simulink model "gm_flyback_pid_vnl"  (R2021b)
settings: Solver=FixedStepDiscrete  StartTime=0.0  StopTime=100e-3  RelTol=1e-3
undefined symbols (not defined in the file or in its folder): DiscIntNeverNeededParam
libraries: simulink x6
Description:
  | Symmetric FIR Filter
  | This example shows how to use HDL Coder(TM) to check, generate,
  | and verify HDL for a fixed-point symmetric FIR filter.
settings Model: Creator=The MathWorks, Inc.  LastModifiedBy=Marco Milanesi
settings SolverCC: AlgebraicLoopSolver=TrustRegion  AutoInsertRateTranBlk=on
settings DataIOCC: LimitDataPoints=on  SaveFormat=Array  SaveOutput=off  SignalLogging=off  SaveTime=off  ReturnWorkspaceOutputs=off  SignalLoggingName=logsOut
settings OptimizationCC: BlockReduction=off  BooleanDataType=off  ConditionallyExecuteInputs=off  DefaultParameterBehavior=Inlined  InheritOutputTypeSmallerThanSingle=on  InlineInvariantSignals=on  ExpressionDepthLimit=2147483647  InitFltsAndDblsToZero=on  LifeSpan=inf  BufferReusableBoundary=off
settings DebuggingCC: AlgebraicLoopMsg=error  SaveWithParameterizedLinksMsg=none  UnderspecifiedInitializationDetection=Classic  MergeDetectMultiDrivingBlocksExec=none  CheckExecutionContextPreStartOutputMsg=on  SignalResolutionControl=TryResolveAllWithWarning  InheritedTsInSrcMsg=none  MultiTaskDSMMsg=warning  MultiTaskCondExecSysMsg=none  SingleTaskRateTransMsg=error  IntegerOverflowMsg=none  ParameterPrecisionLossMsg=none  FcnCallInpInsideContextMsg=warning  BusObjectLabelMismatch=none  StateNameClashWarn=warning  SFUnexpectedBacktrackingDiag=warning  SFNoUnconditionalDefaultTransitionDiag=warning  SFExecutionAtInitializationDiag=none  SFMachineParentedDataDiag=warning  IntegerSaturationMsg=none  ArithmeticOperatorsInVariantConditions=warning
settings HardwareCC: ProdBitPerPointer=32  ProdBitPerSizeT=32  ProdBitPerPtrDiffT=32  ProdLargestAtomicFloat=None  ProdIntDivRoundTo=Undefined  ProdEndianess=Unspecified  ProdWordSize=32  ProdHWDeviceType=ASIC/FPGA  TargetUnknown=on  ProdEqTarget=off
settings ModelReferenceCC: PropagateSignalLabelsOutOfModel=off
settings SFSimCC: SimUseLocalCustomCode=off  CustomCodeUndefinedFunction=UseInterfaceOnly
settings RTWCC: RTWUseLocalCustomCode=off
settings CodeAppCC: StateflowObjectComments=on
settings GRTTargetCC: TargetFcnLib=ansi_tfl_tmw.mat  TargetLangStandard=C89/C90 (ANSI)  CombineOutputUpdateFcns=off  GRTInterface=on
settings ConfigComp: CovMetricSettings=dw  CovSaveCumulativeToWorkspaceVar=on  CovSaveSingleToWorkspaceVar=on  CovExternalEMLEnable=off

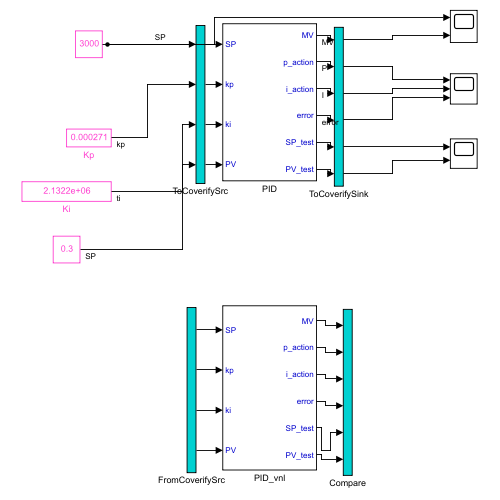
[thumbnail: Simulink's stored preview of the top-level diagram]
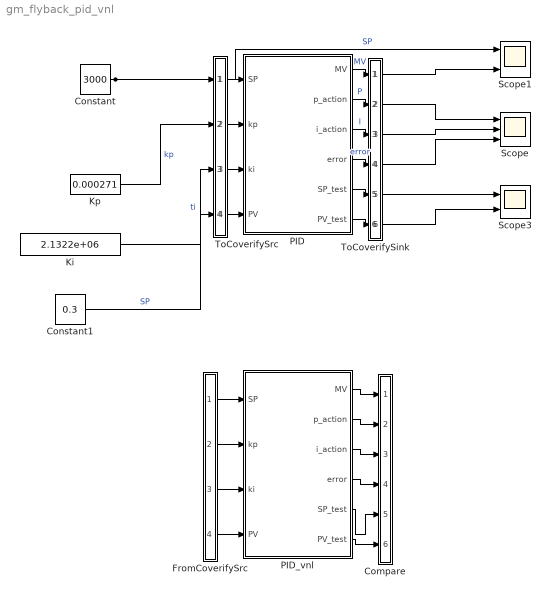
== system gm_flyback_pid_vnl ==
  Compare : Subsystem
      mask Display: disp('')
  Constant : Constant  Value=3000  OutDataTypeStr=fixdt(1,64,32)
  Constant1 : Constant  Value=0.3  OutDataTypeStr=fixdt(1,64,32)
  FromCoverifySrc : Subsystem
      mask Display: disp('')
  Ki : Constant  Value=2.1322e+06  OutDataTypeStr=fixdt(1,64,32)
  Kp : Constant  Value=0.000271  OutDataTypeStr=fixdt(1,64,32)
  PID : Subsystem
  PID_vnl : Subsystem
  Scope : Scope  NumInputPorts=3
  Scope1 : Scope  NumInputPorts=2
  Scope3 : Scope  NumInputPorts=2
  ToCoverifySink : Subsystem
      mask Display: disp('')
  ToCoverifySrc : Subsystem
      mask Display: disp('')
  wires:
  Constant/1 -> Scope1/1, ToCoverifySrc/1(in1)  "SP"
  ToCoverifySrc/1(out1) -> PID/1(SP)
  ToCoverifySrc/2(out2) -> PID/2(kp)
  ToCoverifySrc/3(out3) -> PID/3(ki)
  ToCoverifySrc/4(out4) -> PID/4(PV)
  PID/1(MV) -> ToCoverifySink/1(in1)  "MV"
  PID/2(p_action) -> ToCoverifySink/2(in2)  "P"
  PID/3(i_action) -> ToCoverifySink/3(in3)  "I"
  PID/4(error) -> ToCoverifySink/4(in4)  "error"
  PID/5(SP_test) -> ToCoverifySink/5(in5)
  PID/6(PV_test) -> ToCoverifySink/6(in6)
  Kp/1 -> ToCoverifySrc/2(in2)  "kp"
  Ki/1 -> ToCoverifySrc/3(in3)  "ti"
  Constant1/1 -> ToCoverifySrc/4(in4)  "SP"
  ToCoverifySink/1(out1) -> Scope1/2
  ToCoverifySink/2(out2) -> Scope/1
  ToCoverifySink/3(out3) -> Scope/2
  ToCoverifySink/4(out4) -> Scope/3
  ToCoverifySink/5(out5) -> Scope3/1
  ToCoverifySink/6(out6) -> Scope3/2
  FromCoverifySrc/1(out1) -> PID_vnl/1(SP)
  FromCoverifySrc/2(out2) -> PID_vnl/2(kp)
  FromCoverifySrc/3(out3) -> PID_vnl/3(ki)
  FromCoverifySrc/4(out4) -> PID_vnl/4(PV)
  PID_vnl/1(MV) -> Compare/1(in1)
  PID_vnl/2(p_action) -> Compare/2(in2)
  PID_vnl/3(i_action) -> Compare/3(in3)
  PID_vnl/4(error) -> Compare/4(in4)
  PID_vnl/5(SP_test) -> Compare/5(in5)
  PID_vnl/6(PV_test) -> Compare/6(in6)

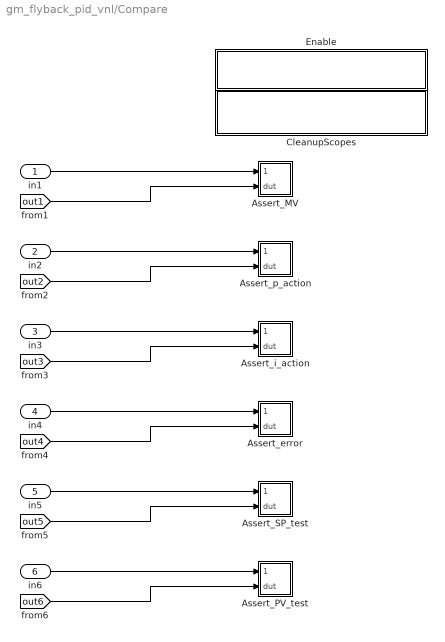
== system gm_flyback_pid_vnl/Compare ==
  in1 : Inport
  in2 : Inport  Port=2
  in3 : Inport  Port=3
  in4 : Inport  Port=4
  in5 : Inport  Port=5
  in6 : Inport  Port=6
  Assert_MV : Subsystem
  Assert_PV_test : Subsystem
  Assert_SP_test : Subsystem
  Assert_error : Subsystem
  Assert_i_action : Subsystem
  Assert_p_action : Subsystem
  CleanupScopes : Subsystem
      settings: OpenFcn=|
      | blkName = gcb; %self block
      | idx = regexp(blkName, '/CleanupScopes$', 'once');
      | blkParent = blkName(1:idx-1);
      | blks=find_system(blkParent, 'LookUnderMasks', 'all','blocktype', 'Scope');
      | for itr = 1:length(blks)
      | 	 hScopeCfg = get_param(blks{itr},'ScopeConfiguration');
      | 	 hScopeCfg.Visible = ~ hScopeCfg.Visible;
      | end
      | drawnow;
      mask Display: fprintf(message('hdlcoder:cosim:vnl_dblclick').getString());
  Enable : Subsystem
      settings: OpenFcn=|
      | blkName = gcb;
      | idx = regexp(blkName, '/Enable$', 'once');
      | blkParent = blkName(1:idx-1);
      | blks=find_system(blkParent, 'LookUnderMasks', 'all','blocktype', 'Assertion');
      | e = get_param(blks{1}, 'Enabled');
      | if strcmp(e, 'on'), f= 'off';, else, f = 'on';, end
      | for ii=1:length(blks), set_param(blks{ii}, 'Enabled', f);, end
      | set_param(gcb, 'MaskDisplay',['fprintf(message(''hdlcoder:cosim:vnl_dblclick_assertions'',','''',upper(e),'''',').getString())']);
      mask Display: fprintf(message('hdlcoder:cosim:vnl_dblclick_assertions','OFF').getString());
  wires:
  in1/1 -> Assert_MV/1(cosim)
  [out1] -> Assert_MV/2(dut)
  in2/1 -> Assert_p_action/1(cosim)
  [out2] -> Assert_p_action/2(dut)
  in3/1 -> Assert_i_action/1(cosim)
  [out3] -> Assert_i_action/2(dut)
  in4/1 -> Assert_error/1(cosim)
  [out4] -> Assert_error/2(dut)
  in5/1 -> Assert_SP_test/1(cosim)
  [out5] -> Assert_SP_test/2(dut)
  in6/1 -> Assert_PV_test/1(cosim)
  [out6] -> Assert_PV_test/2(dut)

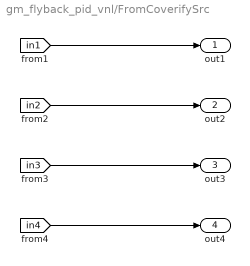
== system gm_flyback_pid_vnl/FromCoverifySrc ==
  out1 : Outport
  out2 : Outport  Port=2
  out3 : Outport  Port=3
  out4 : Outport  Port=4
  wires:
  [in1] -> out1/1
  [in2] -> out2/1
  [in3] -> out3/1
  [in4] -> out4/1

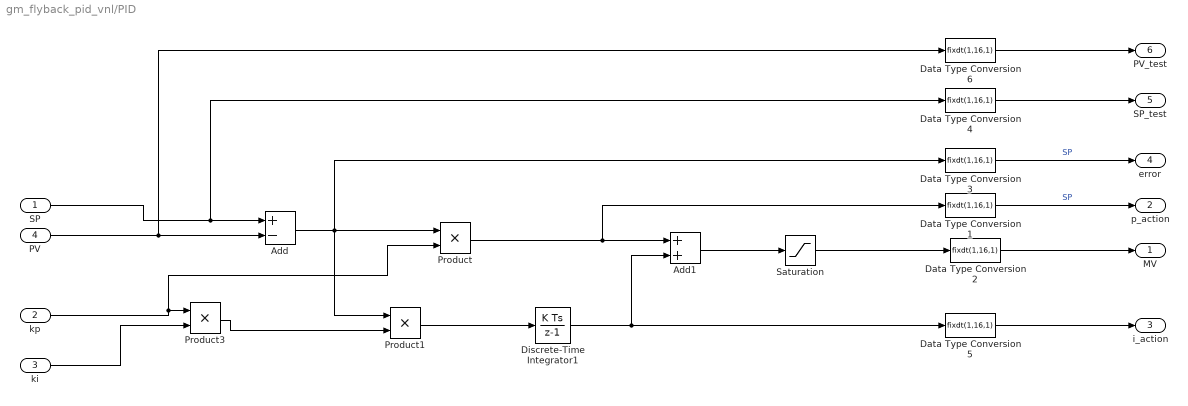
== system gm_flyback_pid_vnl/PID ==
  SP : Inport  OutDataTypeStr=fixdt(1,64,32)  SampleTime=1e-3
  kp : Inport  Port=2  OutDataTypeStr=fixdt(1,64,32)  SampleTime=1e-3
  ki : Inport  Port=3  OutDataTypeStr=fixdt(1,64,32)  SampleTime=1e-3
  PV : Inport  Port=4  OutDataTypeStr=fixdt(1,64,32)  SampleTime=1e-3
  Add : Sum  Inputs=+-  AccumDataTypeStr=fixdt(1,64,32)  OutDataTypeStr=fixdt(1,64,32)
  Add1 : Sum  AccumDataTypeStr=fixdt(1,64,32)  OutDataTypeStr=fixdt(1,64,32)
  Data Type Conversion{1..6} (6 alike) : DataTypeConversion  OutDataTypeStr=fixdt(1,16,1)
  Discrete-Time Integrator1 : DiscreteIntegrator  SampleTime=1e-3  OutDataTypeStr=fixdt(1,64,32)  ICPrevOutput=DiscIntNeverNeededParam  ICPrevScaledInput=DiscIntNeverNeededParam
  Product : Product  OutDataTypeStr=fixdt(1,64,32)
  Product1 : Product  OutDataTypeStr=fixdt(1,64,32)
  Product3 : Product  OutDataTypeStr=fixdt(1,64,32)
  Saturation : Saturate  UpperLimit=255  LowerLimit=0  OutDataTypeStr=fixdt(1,64,32)
  MV : Outport  OutDataTypeStr=fixdt(1,16,1)  SampleTime=1e-3  VectorParamsAs1DForOutWhenUnconnected=off
  p_action : Outport  Port=2  OutDataTypeStr=fixdt(1,16,1)  SampleTime=1e-3  VectorParamsAs1DForOutWhenUnconnected=off
  i_action : Outport  Port=3  OutDataTypeStr=fixdt(1,16,1)  SampleTime=1e-3  VectorParamsAs1DForOutWhenUnconnected=off
  error : Outport  Port=4  OutDataTypeStr=fixdt(1,16,1)  SampleTime=1e-3  VectorParamsAs1DForOutWhenUnconnected=off
  SP_test : Outport  Port=5  OutDataTypeStr=fixdt(1,16,1)  SampleTime=1e-3  VectorParamsAs1DForOutWhenUnconnected=off
  PV_test : Outport  Port=6  OutDataTypeStr=fixdt(1,16,1)  SampleTime=1e-3  VectorParamsAs1DForOutWhenUnconnected=off
  wires:
  kp/1 -> Product/2, Product3/1
  Add1/1 -> Saturation/1
  Product1/1 -> Discrete-Time Integrator1/1
  ki/1 -> Product3/2
  Product3/1 -> Product1/2
  Add/1 -> Data Type Conversion3/1, Product/1, Product1/1
  Product/1 -> Data Type Conversion1/1, Add1/1
  Discrete-Time Integrator1/1 -> Data Type Conversion5/1, Add1/2
  Data Type Conversion1/1 -> p_action/1  "SP"
  Data Type Conversion3/1 -> error/1  "SP"
  Data Type Conversion5/1 -> i_action/1
  Saturation/1 -> Data Type Conversion2/1
  PV/1 -> Data Type Conversion6/1, Add/2
  Data Type Conversion2/1 -> MV/1
  Data Type Conversion4/1 -> SP_test/1
  SP/1 -> Data Type Conversion4/1, Add/1
  Data Type Conversion6/1 -> PV_test/1

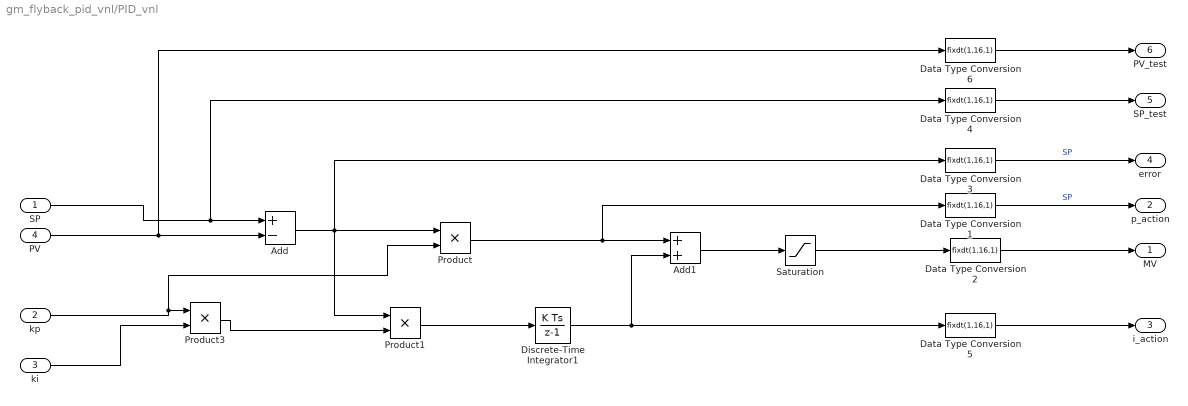
== system gm_flyback_pid_vnl/PID_vnl ==
  SP : Inport  OutDataTypeStr=fixdt(1,64,32)  SampleTime=1e-3
  kp : Inport  Port=2  OutDataTypeStr=fixdt(1,64,32)  SampleTime=1e-3
  ki : Inport  Port=3  OutDataTypeStr=fixdt(1,64,32)  SampleTime=1e-3
  PV : Inport  Port=4  OutDataTypeStr=fixdt(1,64,32)  SampleTime=1e-3
  Add : Sum  Inputs=+-  AccumDataTypeStr=fixdt(1,64,32)  OutDataTypeStr=fixdt(1,64,32)
  Add1 : Sum  AccumDataTypeStr=fixdt(1,64,32)  OutDataTypeStr=fixdt(1,64,32)
  Data Type Conversion{1..6} (6 alike) : DataTypeConversion  OutDataTypeStr=fixdt(1,16,1)
  Discrete-Time Integrator1 : DiscreteIntegrator  SampleTime=1e-3  OutDataTypeStr=fixdt(1,64,32)  ICPrevOutput=DiscIntNeverNeededParam  ICPrevScaledInput=DiscIntNeverNeededParam
  Product : Product  OutDataTypeStr=fixdt(1,64,32)
  Product1 : Product  OutDataTypeStr=fixdt(1,64,32)
  Product3 : Product  OutDataTypeStr=fixdt(1,64,32)
  Saturation : Saturate  UpperLimit=255  LowerLimit=0  OutDataTypeStr=fixdt(1,64,32)
  MV : Outport  OutDataTypeStr=fixdt(1,16,1)  SampleTime=1e-3  VectorParamsAs1DForOutWhenUnconnected=off
  p_action : Outport  Port=2  OutDataTypeStr=fixdt(1,16,1)  SampleTime=1e-3  VectorParamsAs1DForOutWhenUnconnected=off
  i_action : Outport  Port=3  OutDataTypeStr=fixdt(1,16,1)  SampleTime=1e-3  VectorParamsAs1DForOutWhenUnconnected=off
  error : Outport  Port=4  OutDataTypeStr=fixdt(1,16,1)  SampleTime=1e-3  VectorParamsAs1DForOutWhenUnconnected=off
  SP_test : Outport  Port=5  OutDataTypeStr=fixdt(1,16,1)  SampleTime=1e-3  VectorParamsAs1DForOutWhenUnconnected=off
  PV_test : Outport  Port=6  OutDataTypeStr=fixdt(1,16,1)  SampleTime=1e-3  VectorParamsAs1DForOutWhenUnconnected=off
  wires:
  Data Type Conversion6/1 -> PV_test/1
  SP/1 -> Add/1, Data Type Conversion4/1
  Data Type Conversion4/1 -> SP_test/1
  Data Type Conversion2/1 -> MV/1
  PV/1 -> Add/2, Data Type Conversion6/1
  Saturation/1 -> Data Type Conversion2/1
  Data Type Conversion5/1 -> i_action/1
  Data Type Conversion3/1 -> error/1  "SP"
  Data Type Conversion1/1 -> p_action/1  "SP"
  Discrete-Time Integrator1/1 -> Add1/2, Data Type Conversion5/1
  Product/1 -> Add1/1, Data Type Conversion1/1
  Add/1 -> Product1/1, Product/1, Data Type Conversion3/1
  Product3/1 -> Product1/2
  ki/1 -> Product3/2
  Product1/1 -> Discrete-Time Integrator1/1
  Add1/1 -> Saturation/1
  kp/1 -> Product3/1, Product/2

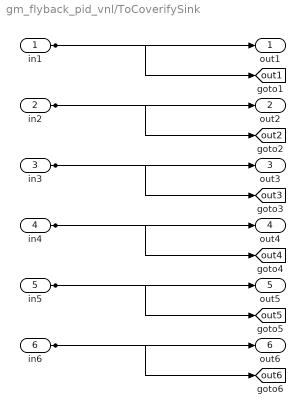
== system gm_flyback_pid_vnl/ToCoverifySink ==
  in1 : Inport
  in2 : Inport  Port=2
  in3 : Inport  Port=3
  in4 : Inport  Port=4
  in5 : Inport  Port=5
  in6 : Inport  Port=6
  out1 : Outport
  out2 : Outport  Port=2
  out3 : Outport  Port=3
  out4 : Outport  Port=4
  out5 : Outport  Port=5
  out6 : Outport  Port=6
  tag scope: out1=global, out2=global, out3=global, out4=global, out5=global, out6=global
  wires:
  in1/1 -> out1/1, [out1]
  in2/1 -> out2/1, [out2]
  in3/1 -> out3/1, [out3]
  in4/1 -> out4/1, [out4]
  in5/1 -> out5/1, [out5]
  in6/1 -> out6/1, [out6]

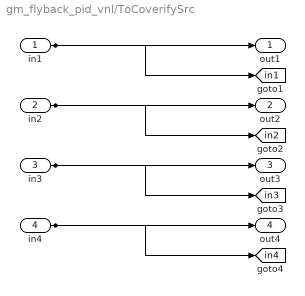
== system gm_flyback_pid_vnl/ToCoverifySrc ==
  in1 : Inport
  in2 : Inport  Port=2
  in3 : Inport  Port=3
  in4 : Inport  Port=4
  out1 : Outport
  out2 : Outport  Port=2
  out3 : Outport  Port=3
  out4 : Outport  Port=4
  tag scope: in1=global, in2=global, in3=global, in4=global
  wires:
  in1/1 -> out1/1, [in1]
  in2/1 -> out2/1, [in2]
  in3/1 -> out3/1, [in3]
  in4/1 -> out4/1, [in4]

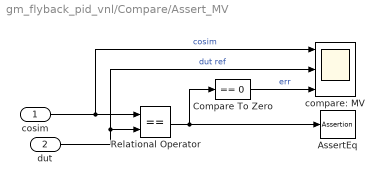
== system gm_flyback_pid_vnl/Compare/Assert_MV ==
  cosim : Inport
  dut : Inport  Port=2
  AssertEq : Assertion  StopWhenAssertionFail=off
  Compare To Zero : simulink/Logic and Bit Operations/Compare To Zero  relop===  OutDataTypeStr=boolean
  Relational Operator : RelationalOperator  Operator===  OutDataTypeStr=boolean  RndMeth=Nearest
  compare: MV : Scope  NumInputPorts=3
  wires:
  Compare To Zero/1 -> compare: MV/3  "err"
  Relational Operator/1 -> Compare To Zero/1, AssertEq/1
  cosim/1 -> compare: MV/1, Relational Operator/1  "cosim"
  dut/1 -> compare: MV/2, Relational Operator/2  "dut ref"

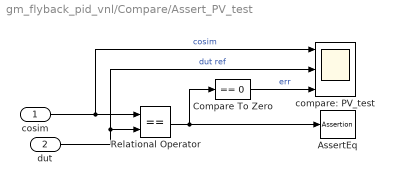
== system gm_flyback_pid_vnl/Compare/Assert_PV_test ==
  cosim : Inport
  dut : Inport  Port=2
  AssertEq : Assertion  StopWhenAssertionFail=off
  Compare To Zero : simulink/Logic and Bit Operations/Compare To Zero  relop===  OutDataTypeStr=boolean
  Relational Operator : RelationalOperator  Operator===  OutDataTypeStr=boolean  RndMeth=Nearest
  compare: PV_test : Scope  NumInputPorts=3
  wires:
  Compare To Zero/1 -> compare: PV_test/3  "err"
  Relational Operator/1 -> Compare To Zero/1, AssertEq/1
  cosim/1 -> compare: PV_test/1, Relational Operator/1  "cosim"
  dut/1 -> compare: PV_test/2, Relational Operator/2  "dut ref"

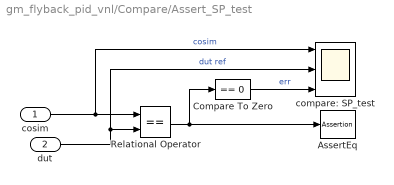
== system gm_flyback_pid_vnl/Compare/Assert_SP_test ==
  cosim : Inport
  dut : Inport  Port=2
  AssertEq : Assertion  StopWhenAssertionFail=off
  Compare To Zero : simulink/Logic and Bit Operations/Compare To Zero  relop===  OutDataTypeStr=boolean
  Relational Operator : RelationalOperator  Operator===  OutDataTypeStr=boolean  RndMeth=Nearest
  compare: SP_test : Scope  NumInputPorts=3
  wires:
  Compare To Zero/1 -> compare: SP_test/3  "err"
  Relational Operator/1 -> Compare To Zero/1, AssertEq/1
  cosim/1 -> compare: SP_test/1, Relational Operator/1  "cosim"
  dut/1 -> compare: SP_test/2, Relational Operator/2  "dut ref"

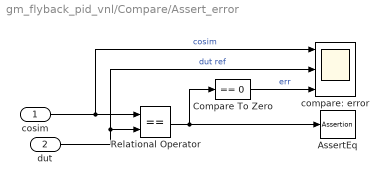
== system gm_flyback_pid_vnl/Compare/Assert_error ==
  cosim : Inport
  dut : Inport  Port=2
  AssertEq : Assertion  StopWhenAssertionFail=off
  Compare To Zero : simulink/Logic and Bit Operations/Compare To Zero  relop===  OutDataTypeStr=boolean
  Relational Operator : RelationalOperator  Operator===  OutDataTypeStr=boolean  RndMeth=Nearest
  compare: error : Scope  NumInputPorts=3
  wires:
  Compare To Zero/1 -> compare: error/3  "err"
  Relational Operator/1 -> Compare To Zero/1, AssertEq/1
  cosim/1 -> compare: error/1, Relational Operator/1  "cosim"
  dut/1 -> compare: error/2, Relational Operator/2  "dut ref"

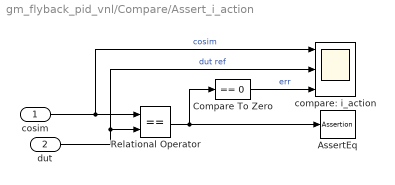
== system gm_flyback_pid_vnl/Compare/Assert_i_action ==
  cosim : Inport
  dut : Inport  Port=2
  AssertEq : Assertion  StopWhenAssertionFail=off
  Compare To Zero : simulink/Logic and Bit Operations/Compare To Zero  relop===  OutDataTypeStr=boolean
  Relational Operator : RelationalOperator  Operator===  OutDataTypeStr=boolean  RndMeth=Nearest
  compare: i_action : Scope  NumInputPorts=3
  wires:
  Compare To Zero/1 -> compare: i_action/3  "err"
  Relational Operator/1 -> Compare To Zero/1, AssertEq/1
  cosim/1 -> compare: i_action/1, Relational Operator/1  "cosim"
  dut/1 -> compare: i_action/2, Relational Operator/2  "dut ref"

== system gm_flyback_pid_vnl/Compare/Assert_p_action ==
  cosim : Inport
  dut : Inport  Port=2
  AssertEq : Assertion  StopWhenAssertionFail=off
  Compare To Zero : simulink/Logic and Bit Operations/Compare To Zero  relop===  OutDataTypeStr=boolean
  Relational Operator : RelationalOperator  Operator===  OutDataTypeStr=boolean  RndMeth=Nearest
  compare: p_action : Scope  NumInputPorts=3
  wires:
  Compare To Zero/1 -> compare: p_action/3  "err"
  Relational Operator/1 -> Compare To Zero/1, AssertEq/1
  cosim/1 -> compare: p_action/1, Relational Operator/1  "cosim"
  dut/1 -> compare: p_action/2, Relational Operator/2  "dut ref"

== system gm_flyback_pid_vnl/Compare/CleanupScopes ==

== system gm_flyback_pid_vnl/Compare/Enable ==
